simulink subsystem "extractEsdStats"  (R2021a)
settings: Solver=VariableStepAuto  StartTime=0.0  StopTime=10.0  RelTol=1e-3
undefined symbols (not defined in the file or in its folder): Newton, Raphson
settings Model: Creator=trevor  LastModifiedBy=trevor
settings SolverCC: AlgebraicLoopSolver=TrustRegion
settings DebuggingCC: SFMachineParentedDataDiag=warning

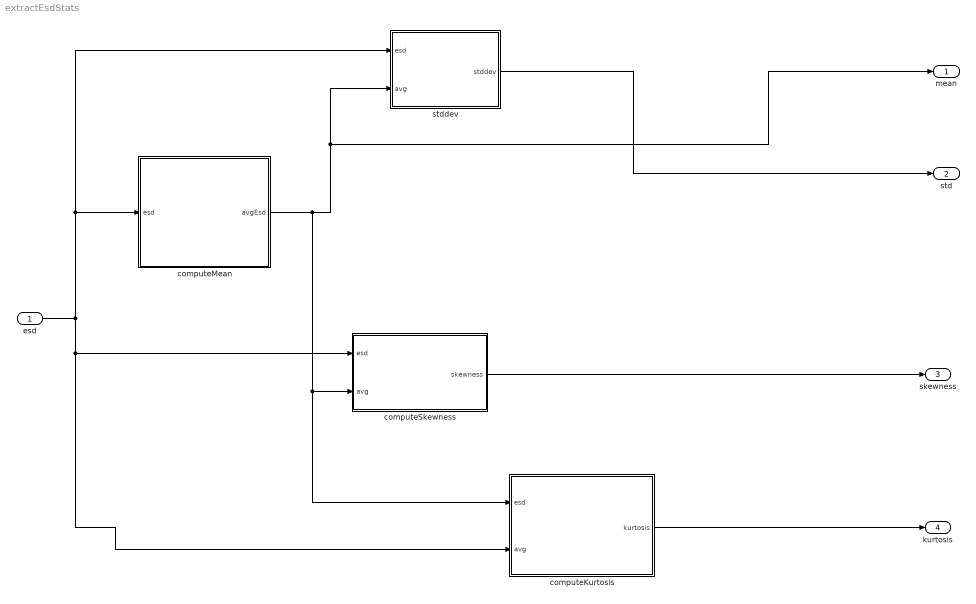
== system extractEsdStats ==
  esd : Inport
  computeKurtosis : Subsystem
  computeMean : Subsystem
  computeSkewness : Subsystem
  stddev : Subsystem
  mean : Outport
  std : Outport  Port=2
  skewness : Outport  Port=3
  kurtosis : Outport  Port=4
  wires:
  stddev/1(stddev) -> std/1
  esd/1 -> stddev/1(esd), computeMean/1(esd), computeSkewness/1(esd), computeKurtosis/2(avg)
  computeKurtosis/1(kurtosis) -> kurtosis/1
  computeSkewness/1(skewness) -> skewness/1
  computeMean/1(avgEsd) -> stddev/2(avg), mean/1, computeKurtosis/1(esd), computeSkewness/2(avg)

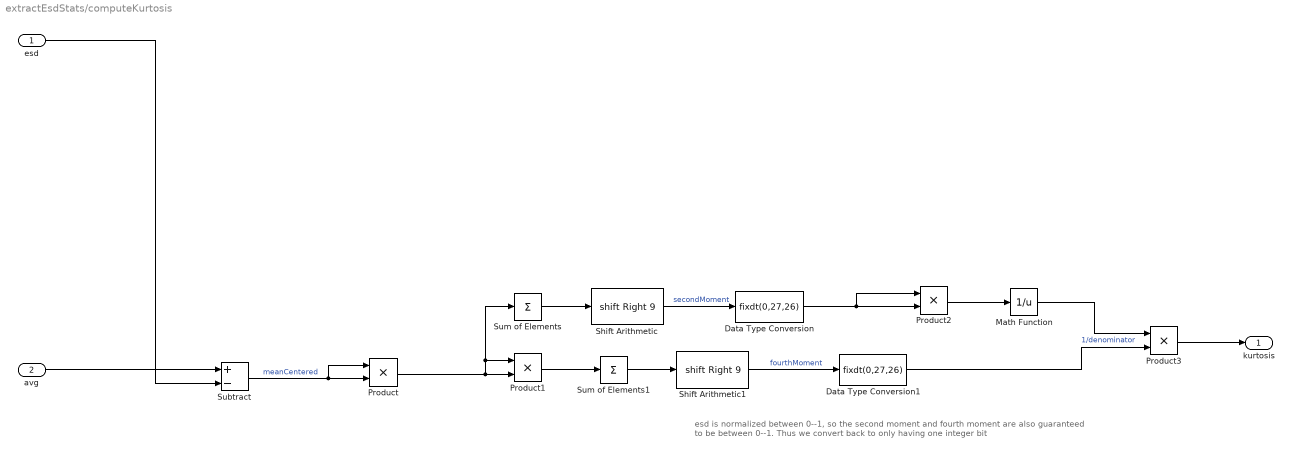
== system extractEsdStats/computeKurtosis ==
  note: esd is normalized between 0--1, so the second moment and fourth moment are also guaranteed to be between 0--1. Thus we convert back to only having one integer bit
  esd : Inport
  avg : Inport  Port=2
  Data Type Conversion : DataTypeConversion  OutDataTypeStr=fixdt(0,27,26)
  Data Type Conversion1 : DataTypeConversion  OutDataTypeStr=fixdt(0,27,26)
  Math Function : Math  Operator=reciprocal  OutDataTypeStr=fixdt(0,42,16)  RndMeth=Zero  SaturateOnIntegerOverflow=on
  Product : Product  OutDataTypeStr=fixdt(0,27,26)
  Product1 : Product  OutDataTypeStr=Inherit: Same as first input
  Product2 : Product  OutDataTypeStr=Inherit: Same as first input
  Product3 : Product  OutDataTypeStr=Inherit: Match scaling
  Shift Arithmetic : ArithShift  BitShiftNumber=9  BitShiftDirection=Right
  Shift Arithmetic1 : ArithShift  BitShiftNumber=9  BitShiftDirection=Right
  Subtract : Sum  Inputs=+-
  Sum of Elements : Sum  Inputs=+
  Sum of Elements1 : Sum  Inputs=+
  kurtosis : Outport
  wires:
  Data Type Conversion1/1 -> Product3/2
  Data Type Conversion/1 -> Product2/2, Product2/1
  Math Function/1 -> Product3/1  "1/denominator"
  Sum of Elements/1 -> Shift Arithmetic/1
  Product/1 -> Product1/2, Product1/1, Sum of Elements/1
  Sum of Elements1/1 -> Shift Arithmetic1/1
  Shift Arithmetic/1 -> Data Type Conversion/1  "secondMoment"
  avg/1 -> Subtract/1
  esd/1 -> Subtract/2
  Product3/1 -> kurtosis/1
  Product1/1 -> Sum of Elements1/1
  Subtract/1 -> Product/2, Product/1  "meanCentered"
  Shift Arithmetic1/1 -> Data Type Conversion1/1  "fourthMoment"
  Product2/1 -> Math Function/1

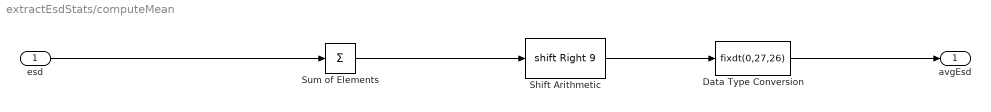
== system extractEsdStats/computeMean ==
  esd : Inport
  Data Type Conversion : DataTypeConversion  OutDataTypeStr=fixdt(0,27,26)
  Shift Arithmetic : ArithShift  BitShiftNumber=9  BitShiftDirection=Right
  Sum of Elements : Sum  Inputs=+
  avgEsd : Outport
  wires:
  Data Type Conversion/1 -> avgEsd/1
  Sum of Elements/1 -> Shift Arithmetic/1
  esd/1 -> Sum of Elements/1
  Shift Arithmetic/1 -> Data Type Conversion/1

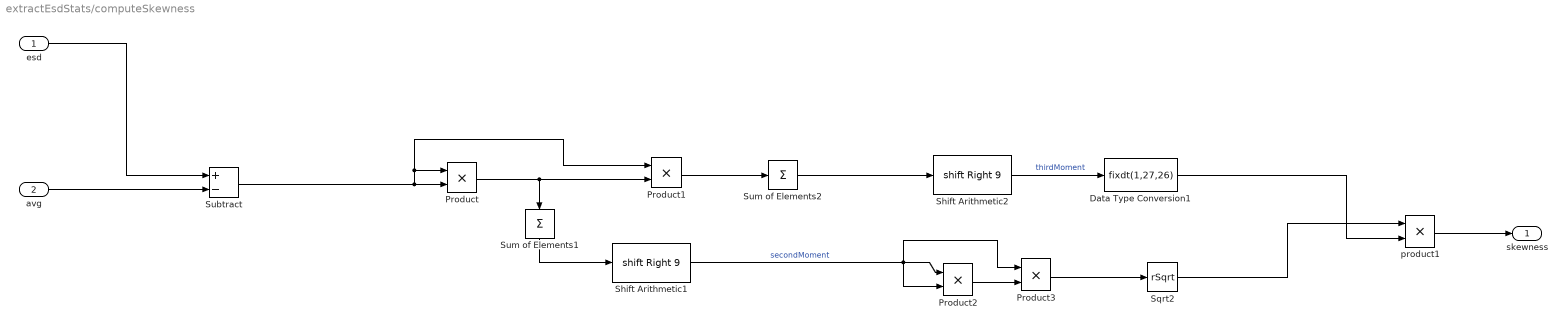
== system extractEsdStats/computeSkewness ==
  esd : Inport
  avg : Inport  Port=2
  Data Type Conversion1 : DataTypeConversion  OutDataTypeStr=fixdt(1,27,26)
  Product : Product  OutMin=0  OutMax=1  OutDataTypeStr=fixdt(0,40,39)
  Product1 : Product  OutDataTypeStr=Inherit: Same as first input
  Product2 : Product  OutDataTypeStr=Inherit: Same as first input
  Product3 : Product  OutDataTypeStr=Inherit: Same as first input
  Shift Arithmetic1 : ArithShift  BitShiftNumber=9  BitShiftDirection=Right
  Shift Arithmetic2 : ArithShift  BitShiftNumber=9  BitShiftDirection=Right
  Sqrt2 : Sqrt  Operator=rSqrt  AlgorithmType=Newton-Raphson  Iterations=10  SaturateOnIntegerOverflow=on  OutDataTypeStr=Inherit: Inherit via internal rule
  Subtract : Sum  Inputs=+-
  Sum of Elements1 : Sum  Inputs=+
  Sum of Elements2 : Sum  Inputs=+
  product1 : Product  Inputs=**  RndMeth=Zero  SaturateOnIntegerOverflow=on
  skewness : Outport
  wires:
  Product2/1 -> Product3/2
  Product3/1 -> Sqrt2/1
  Data Type Conversion1/1 -> product1/2
  Sqrt2/1 -> product1/1
  Subtract/1 -> Product/2, Product/1, Product1/1
  Sum of Elements2/1 -> Shift Arithmetic2/1
  Sum of Elements1/1 -> Shift Arithmetic1/1
  product1/1 -> skewness/1
  Shift Arithmetic2/1 -> Data Type Conversion1/1  "thirdMoment"
  Shift Arithmetic1/1 -> Product2/1, Product3/1, Product2/2  "secondMoment"
  Product1/1 -> Sum of Elements2/1
  Product/1 -> Product1/2, Sum of Elements1/1
  avg/1 -> Subtract/2
  esd/1 -> Subtract/1

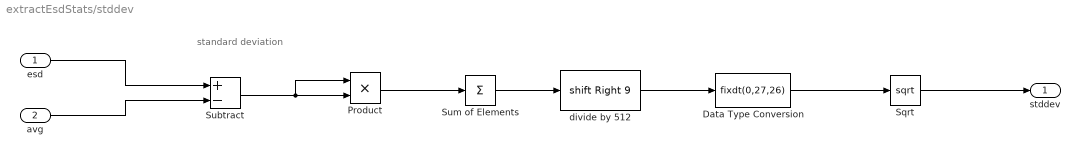
== system extractEsdStats/stddev ==
  note: standard deviation
  esd : Inport
  avg : Inport  Port=2
  Data Type Conversion : DataTypeConversion  OutDataTypeStr=fixdt(0,27,26)
  Product : Product  OutDataTypeStr=fixdt(0,27,26)
  Sqrt : Sqrt  SaturateOnIntegerOverflow=on
  Subtract : Sum  Inputs=+-  OutDataTypeStr=Inherit: Same as accumulator
  Sum of Elements : Sum  Inputs=+
  divide by 512 : ArithShift  BitShiftNumber=9  BitShiftDirection=Right
  stddev : Outport
  wires:
  Sum of Elements/1 -> divide by 512/1
  esd/1 -> Subtract/1
  Sqrt/1 -> stddev/1
  Subtract/1 -> Product/2, Product/1
  avg/1 -> Subtract/2
  divide by 512/1 -> Data Type Conversion/1
  Product/1 -> Sum of Elements/1
  Data Type Conversion/1 -> Sqrt/1
